simulink model "Aquisition"  (R2014a)
settings: Solver=ode3  StartTime=0.0  StopTime=60  FixedStep=1/1000  RelTol=1e-3
undefined symbols (not defined in the file or in its folder): National_Instruments, PCI, pin
libraries: rtwinlib x1
settings Model: SimulationMode=external  ExtModeTrigDuration=100000  Creator=betojr  LastModifiedBy=unieerisantos
settings HardwareCC: ProdIntDivRoundTo=Zero  ProdEndianess=LittleEndian  ProdHWDeviceType=Generic->32-bit x86 compatible
settings RTWCC: SystemTargetFile=rtwin.tlc  TemplateMakefile=rtwin.tmf  Description=Real-Time Windows Target  ProcessScript=rtwin_make_rtw_hook  RTWCompilerOptimization=On
settings CodeAppCC: MaxIdLength=95
settings RTWinTargetCC: TargetLibSuffix=_rtwin.lib  TargetPreCompLibLocation=C:\Program Files\MATLAB\R2014a\toolbox\rtw\targets\rtwin\lib\win64

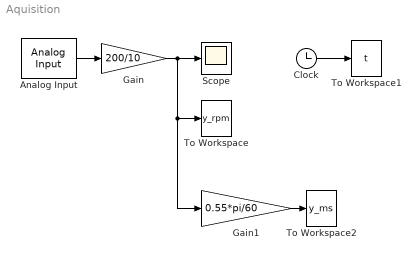
== system Aquisition ==
  Analog Input : rtwinlib/Analog Input  SampleTime=1/1000  MaxMissedTicks=10  ShowMissedTicks=off  YieldWhenWaiting=off  DrvName=National_Instruments/PCI-6221_37-pin  DrvAddress=4294967295  DrvOptions=[0 0 0 0 0]  Channels=1  RangeMode=1  VoltRange=1  DataType=1
      settings: AttributesFormatString=National Instruments\nPCI-6221 37-pin [auto]
  Clock : Clock
  Gain : Gain  Gain=200/10
  Gain1 : Gain  Gain=0.55*pi/60
  Scope : Scope
      settings: TimeRange=60  YMin=0  YMax=75
  To Workspace : ToWorkspace  VariableName=y_rpm  SampleTime=-1
  To Workspace1 : ToWorkspace  VariableName=t  SampleTime=-1
  To Workspace2 : ToWorkspace  VariableName=y_ms  SampleTime=-1
  wires:
  Analog Input/1 -> Gain/1
  Clock/1 -> To Workspace1/1
  Gain/1 -> Gain1/1, To Workspace/1, Scope/1
  Gain1/1 -> To Workspace2/1
